simulink model "dynamics_block"  (R2022b)
settings: Solver=VariableStepAuto  StartTime=0.0  StopTime=10.0  RelTol=1e-3
settings Model: Creator=lasto  LastModifiedBy=lasto

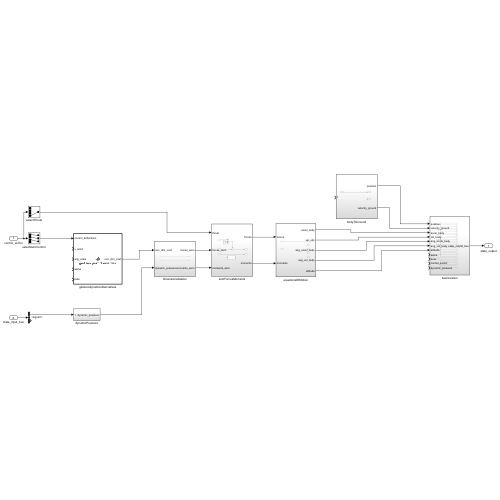
[thumbnail: Simulink's stored preview of the top-level diagram]
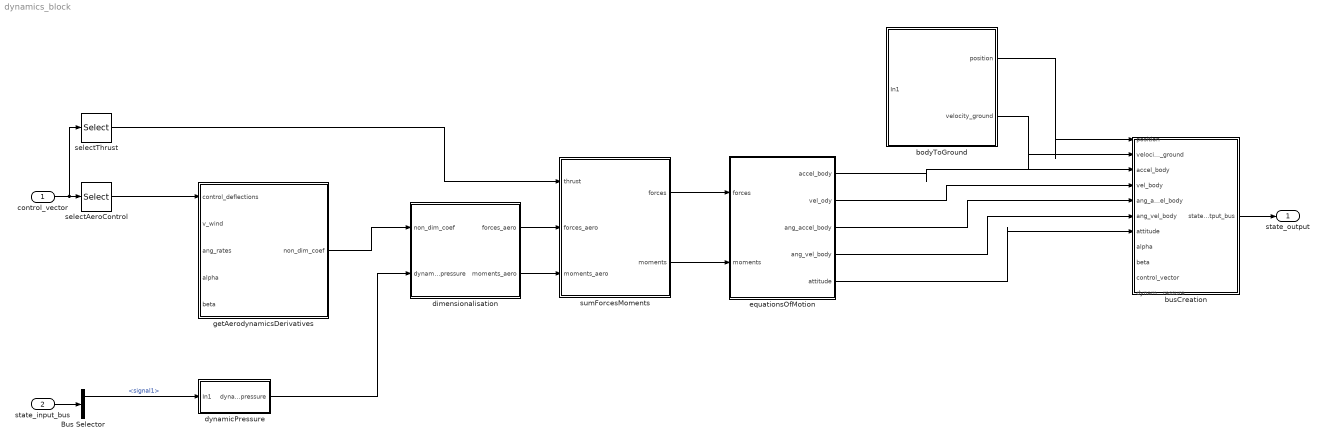
== system dynamics_block ==
  control_vector : Inport
  state_input_bus : Inport  Port=2
  Bus Selector : BusSelector  OutputSignals=signal1,signal2
  bodyToGround : Subsystem
  busCreation : Subsystem
  dimensionalisation : Subsystem
  dynamicPressure : Subsystem
  equationsOfMotion : Subsystem
  getAerodynamicsDerivatives : MATLAB Function  TreatAsAtomicUnit=on
  selectAeroControl : Selector  InputPortWidth=4  IndexOptions=Index vector (dialog)  Indices=[1 2 3]  OutputSizes=1
  selectThrust : Selector  InputPortWidth=4  IndexOptions=Index vector (dialog)  Indices=[4]  OutputSizes=1
  sumForcesMoments : Subsystem
  state_output : Outport
  wires:
  control_vector/1 -> selectThrust/1, selectAeroControl/1
  sumForcesMoments/2(moments) -> equationsOfMotion/2(moments)
  sumForcesMoments/1(forces) -> equationsOfMotion/1(forces)
  dimensionalisation/1(forces_aero) -> sumForcesMoments/2(forces_aero)
  Bus Selector/1 -> dynamicPressure/1(In1)  "<signal1>"
  selectAeroControl/1 -> getAerodynamicsDerivatives/1(control_deflections)
  getAerodynamicsDerivatives/1(non_dim_coef) -> dimensionalisation/1(non_dim_coef)
  dynamicPressure/1(dynamic_pressure) -> dimensionalisation/2(dynamic_pressure)
  busCreation/1(state_output_bus) -> state_output/1
  selectThrust/1 -> sumForcesMoments/1(thrust)
  dimensionalisation/2(moments_aero) -> sumForcesMoments/3(moments_aero)
  state_input_bus/1 -> Bus Selector/1
  bodyToGround/1(position) -> busCreation/1(position)
  equationsOfMotion/1(accel_body) -> busCreation/3(accel_body)
  equationsOfMotion/2(vel_ody) -> busCreation/4(vel_body)
  equationsOfMotion/3(ang_accel_body) -> busCreation/5(ang_accel_body)
  equationsOfMotion/4(ang_vel_body) -> busCreation/6(ang_vel_body)
  bodyToGround/2(velocity_ground) -> busCreation/2(velocity_ground)
  equationsOfMotion/5(attitude) -> busCreation/7(attitude)

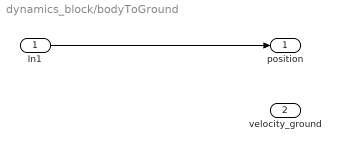
== system dynamics_block/bodyToGround ==
  In1 : Inport
  position : Outport
  velocity_ground : Outport  Port=2
  wires:
  In1/1 -> position/1

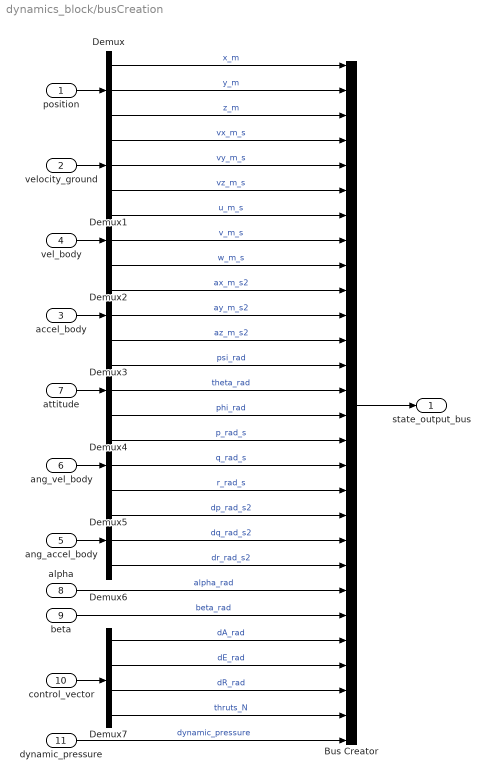
== system dynamics_block/busCreation ==
  position : Inport
  velocity_ground : Inport  Port=2
  accel_body : Inport  Port=3
  vel_body : Inport  Port=4
  ang_accel_body : Inport  Port=5
  ang_vel_body : Inport  Port=6
  attitude : Inport  Port=7
  alpha : Inport  Port=8
  beta : Inport  Port=9
  control_vector : Inport  Port=10
  dynamic_pressure : Inport  Port=11
  Bus Creator : BusCreator  Inputs=28
  Demux{,1..6} (7 alike) : Demux  Outputs=3
  Demux7 : Demux
  state_output_bus : Outport
  wires:
  position/1 -> Demux/1
  Bus Creator/1 -> state_output_bus/1
  Demux/1 -> Bus Creator/1  "x_m"
  Demux/2 -> Bus Creator/2  "y_m"
  Demux/3 -> Bus Creator/3  "z_m"
  Demux1/1 -> Bus Creator/4  "vx_m_s"
  Demux1/2 -> Bus Creator/5  "vy_m_s"
  Demux1/3 -> Bus Creator/6  "vz_m_s"
  Demux2/1 -> Bus Creator/7  "u_m_s"
  Demux2/2 -> Bus Creator/8  "v_m_s"
  Demux2/3 -> Bus Creator/9  "w_m_s"
  Demux3/1 -> Bus Creator/10  "ax_m_s2"
  Demux3/2 -> Bus Creator/11  "ay_m_s2"
  Demux3/3 -> Bus Creator/12  "az_m_s2"
  Demux4/1 -> Bus Creator/13  "psi_rad"
  Demux4/2 -> Bus Creator/14  "theta_rad"
  Demux4/3 -> Bus Creator/15  "phi_rad"
  Demux5/1 -> Bus Creator/16  "p_rad_s"
  Demux5/3 -> Bus Creator/18  "r_rad_s"
  Demux5/2 -> Bus Creator/17  "q_rad_s"
  Demux6/1 -> Bus Creator/19  "dp_rad_s2"
  Demux6/2 -> Bus Creator/20  "dq_rad_s2"
  Demux6/3 -> Bus Creator/21  "dr_rad_s2"
  velocity_ground/1 -> Demux1/1
  vel_body/1 -> Demux2/1
  accel_body/1 -> Demux3/1
  attitude/1 -> Demux4/1
  ang_vel_body/1 -> Demux5/1
  ang_accel_body/1 -> Demux6/1
  alpha/1 -> Bus Creator/22  "alpha_rad"
  beta/1 -> Bus Creator/23  "beta_rad"
  Demux7/1 -> Bus Creator/24  "dA_rad"
  Demux7/2 -> Bus Creator/25  "dE_rad"
  Demux7/3 -> Bus Creator/26  "dR_rad"
  control_vector/1 -> Demux7/1
  dynamic_pressure/1 -> Bus Creator/28  "dynamic_pressure"
  Demux7/4 -> Bus Creator/27  "thruts_N"

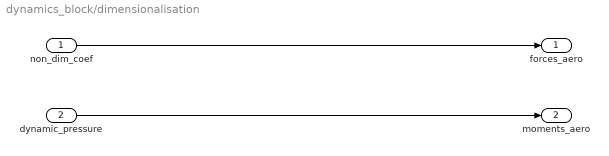
== system dynamics_block/dimensionalisation ==
  non_dim_coef : Inport
  dynamic_pressure : Inport  Port=2
  forces_aero : Outport
  moments_aero : Outport  Port=2
  wires:
  non_dim_coef/1 -> forces_aero/1
  dynamic_pressure/1 -> moments_aero/1

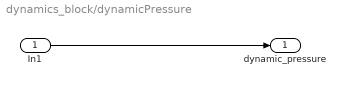
== system dynamics_block/dynamicPressure ==
  In1 : Inport
  dynamic_pressure : Outport
  wires:
  In1/1 -> dynamic_pressure/1

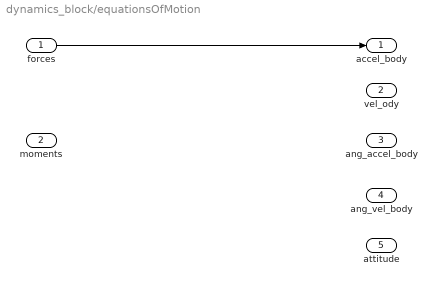
== system dynamics_block/equationsOfMotion ==
  forces : Inport
  moments : Inport  Port=2
  accel_body : Outport
  vel_ody : Outport  Port=2
  ang_accel_body : Outport  Port=3
  ang_vel_body : Outport  Port=4
  attitude : Outport  Port=5
  wires:
  forces/1 -> accel_body/1

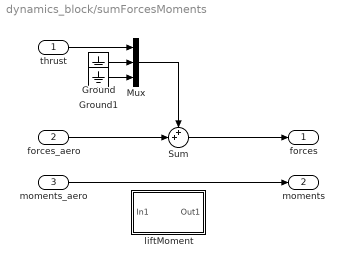
== system dynamics_block/sumForcesMoments ==
  thrust : Inport
  forces_aero : Inport  Port=2
  moments_aero : Inport  Port=3
  Ground : Ground
  Ground1 : Ground
  Mux : Mux  Inputs=3
  Sum : Sum  Inputs=++|
  liftMoment : Subsystem
  forces : Outport
  moments : Outport  Port=2
  wires:
  forces_aero/1 -> Sum/2
  moments_aero/1 -> moments/1
  thrust/1 -> Mux/1
  Ground/1 -> Mux/2
  Ground1/1 -> Mux/3
  Sum/1 -> forces/1
  Mux/1 -> Sum/1

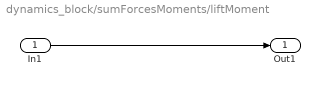
== system dynamics_block/sumForcesMoments/liftMoment ==
  In1 : Inport
  Out1 : Outport
  wires:
  In1/1 -> Out1/1

== matlab function dynamics_block/getAerodynamicsDerivatives ==
  data: control_deflections input; v_wind input; non_dim_coef output; ang_rates input; alpha input; beta input
function non_dim_coef  = getAerodynamicDerivatives(control_deflections,v_wind,ang_rates,alpha,beta)



end
